simulink model "es3"  (R2021a)
settings: Solver=VariableStepAuto  StartTime=0.0  StopTime=10.0  RelTol=1e-3
settings Model: Creator=bonvoltnuovo  LastModifiedBy=bonvoltnuovo

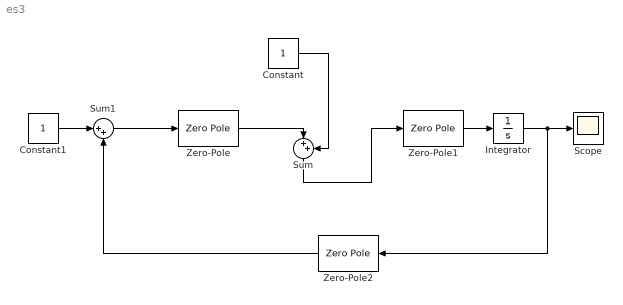
== system es3 ==
  Constant : Constant
  Constant1 : Constant
  Integrator : Integrator
  Scope : Scope
  Sum : Sum  Inputs=|++
  Sum1 : Sum  Inputs=|++
  Zero-Pole : ZeroPole  Zeros=[0.75]  Poles=[1]
  Zero-Pole1 : ZeroPole  Zeros=[5.2]  Poles=[0.03 1]
  Zero-Pole2 : ZeroPole  Zeros=[9.87e04 0]  Poles=[1 444.3 9.87e04]
  wires:
  Zero-Pole/1 -> Sum/1
  Constant/1 -> Sum/2
  Sum/1 -> Zero-Pole1/1
  Zero-Pole1/1 -> Integrator/1
  Sum1/1 -> Zero-Pole/1
  Zero-Pole2/1 -> Sum1/2
  Integrator/1 -> Scope/1, Zero-Pole2/1
  Constant1/1 -> Sum1/1
